simulink model "bench_flat"  (R2025b)
settings: Solver=ode4  StartTime=0.0  StopTime=inf  FixedStep=Ts_gcs  RelTol=1e-3
InitFcn:
  | bench_init_fcn(mocap);
undefined symbols (not defined in the file): mocap, Ts_gcs
libraries: instrumentseriallib x2, sldrtlib x1
Description:
  | Four-drone ground station of the FLATNESS variant (mirror of bench.slx).
  | MotiveMocapMulti streams every rigid body in mocap.streaming_ids, one gcu_flat instance
  | per entry (model argument drone_idx = slice of the shared traj built by bench_init_fcn).
  | Each path packs its own 106-byte flat frame; the four frames are concatenated into one
  | 424-byte USB frame, and gcs_sender_flat forwards the freshest frame per id.
  | Swarm mode: params; ref = swarm_precompute(...); init_trajectory_swarm(id) per drone; Run.
  | Evaluation: flight_evaluation_flat(id).
settings Model: DataDictionary=project.sldd  SimulationMode=accelerator  Creator=Nick  LastModifiedBy=Rakete
settings SolverCC: AutoInsertRateTranBlk=on

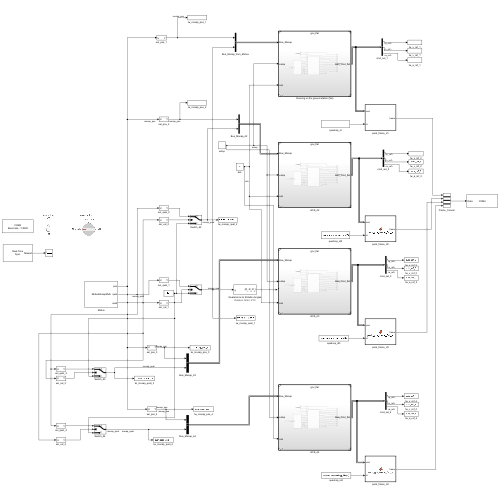
[thumbnail: Simulink's stored preview of the top-level diagram]
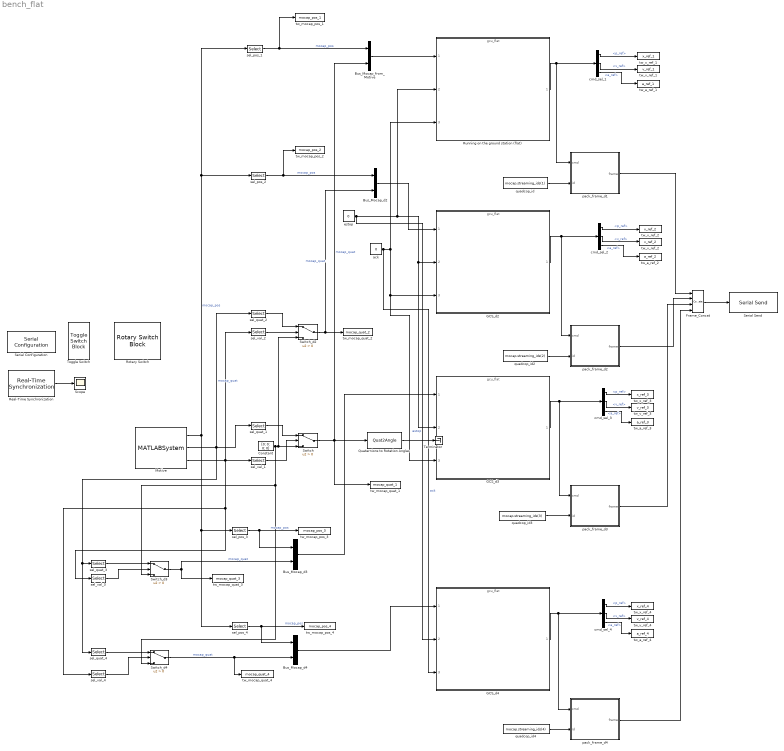
== system bench_flat ==
  Bus_Mocap_d2 : BusCreator  Inputs=2  OutDataTypeStr=Bus: Bus_Mocap
  Bus_Mocap_d3 : BusCreator  Inputs=2  OutDataTypeStr=Bus: Bus_Mocap
  Bus_Mocap_d4 : BusCreator  Inputs=2  OutDataTypeStr=Bus: Bus_Mocap
  Bus_Mocap_from_Motive : BusCreator  Inputs=2  OutDataTypeStr=Bus: Bus_Mocap
  Constant : Constant  Value=[0; 0; 0; 0]
  Frame_Concat : Concatenate  NumInputs=4
  GCS_d2 : ModelReference  ModelNameDialog=gcu_flat  ParameterArgumentNames=drone_idx  ParameterArgumentValues=2  UsingDefaultArgumentValue=0  SimulationMode=Normal  ModelReferenceVersion=1.330
  GCS_d3 : ModelReference  ModelNameDialog=gcu_flat  ParameterArgumentNames=drone_idx  ParameterArgumentValues=3  UsingDefaultArgumentValue=0  SimulationMode=Normal  ModelReferenceVersion=1.330
  GCS_d4 : ModelReference  ModelNameDialog=gcu_flat  ParameterArgumentNames=drone_idx  ParameterArgumentValues=4  UsingDefaultArgumentValue=0  SimulationMode=Normal  ModelReferenceVersion=1.330
  Motive : MATLABSystem  System=MotiveMocapMulti  HostIP=mocap.host_ip  ClientIP=mocap.client_ip  StreamingIDs=mocap.streaming_ids  SampleTimeSec=Ts_gcs  Verbose=on
      mask Type: MotiveMocapMulti
  Quaternions to Rotation Angles : Quat2Angle
      settings: AttributesFormatString=Rotation Order: %<rotationOrder>
  Real-Time Synchronization : sldrtlib/Real-Time Synchronization  SampleTime=Ts_gcs  MaxMissedTicks=inf  ShowMissedTicks=on  YieldWhenWaiting=off
  Rotary Switch : RotarySwitchBlock
  Running on the ground station (flat) : ModelReference  ModelNameDialog=gcu_flat  ParameterArgumentNames=drone_idx  ParameterArgumentValues=1  UsingDefaultArgumentValue=0  SimulationMode=Normal  ModelReferenceVersion=1.330
  Scope : Scope
      settings: ActiveDisplayYMinimum=-1  ActiveDisplayYMaximum=1
  Serial Configuration : instrumentseriallib/Serial Configuration  Priority=-200000  PortSel=COM4  Port=COM4  ComPort=COM4  BaudRate=115200  DataBits=8  Parity=none  StopBits=1  ByteOrder=little-endian  FlowControl=none  Timeout=10  SimulateUsing=Interpreted execution  BlockInModel=on  aMode=1
      settings: LibrarySourceBlock=c2000lib/Host Communication/Serial Configuration
  Serial Send : instrumentseriallib/Serial Send  Priority=1  PortSel=COM4  Port=COM4  ComPort=COM4  Header=[]  Terminator=<none>  CustomTerminator=[]  EnableBlockingMode=on  SimulateUsing=Interpreted execution  BlockInModel=on  aMode=1
      settings: LibrarySourceBlock=c2000lib/Host Communication/Serial Send
  Switch : Switch  Criteria=u2 > Threshold  SaturateOnIntegerOverflow=off  InputSameDT=off
  Switch_d2 : Switch  Criteria=u2 > Threshold  SaturateOnIntegerOverflow=off  InputSameDT=off
  Switch_d3 : Switch  Criteria=u2 > Threshold  SaturateOnIntegerOverflow=off  InputSameDT=off
  Switch_d4 : Switch  Criteria=u2 > Threshold  SaturateOnIntegerOverflow=off  InputSameDT=off
  Terminator : Terminator
  Toggle Switch : ToggleSwitchBlock
  ack : Constant  Value=0  OutDataTypeStr=boolean
  cmd_sel_{1..4} (4 alike) : BusSelector  OutputSignals=p_ref,v_ref,a_ref
  estop : Constant  Value=0  OutDataTypeStr=uint8
  pack_frame_d1 : MATLAB Function  TreatAsAtomicUnit=on
  pack_frame_d2 : MATLAB Function  TreatAsAtomicUnit=on
  pack_frame_d3 : MATLAB Function  TreatAsAtomicUnit=on
  pack_frame_d4 : MATLAB Function  TreatAsAtomicUnit=on
  quadcop_id : Constant  Value=mocap.streaming_ids(1)  OutDataTypeStr=uint8
  quadcop_id2 : Constant  Value=mocap.streaming_ids(2)  OutDataTypeStr=uint8
  quadcop_id3 : Constant  Value=mocap.streaming_ids(3)  OutDataTypeStr=uint8
  quadcop_id4 : Constant  Value=mocap.streaming_ids(4)  OutDataTypeStr=uint8
  sel_pos_1 : Selector  NumberOfDimensions=2  IndexOptions=Select all,Index vector (dialog)  Indices=1,1  OutputSizes=1
  sel_pos_2 : Selector  NumberOfDimensions=2  IndexOptions=Select all,Index vector (dialog)  Indices=1,2  OutputSizes=1
  sel_pos_3 : Selector  NumberOfDimensions=2  IndexOptions=Select all,Index vector (dialog)  Indices=1,3  OutputSizes=1
  sel_pos_4 : Selector  NumberOfDimensions=2  IndexOptions=Select all,Index vector (dialog)  Indices=1,4  OutputSizes=1
  sel_quat_1 : Selector  NumberOfDimensions=2  IndexOptions=Select all,Index vector (dialog)  Indices=1,1  OutputSizes=1
  sel_quat_2 : Selector  NumberOfDimensions=2  IndexOptions=Select all,Index vector (dialog)  Indices=1,2  OutputSizes=1
  sel_quat_3 : Selector  NumberOfDimensions=2  IndexOptions=Select all,Index vector (dialog)  Indices=1,3  OutputSizes=1
  sel_quat_4 : Selector  NumberOfDimensions=2  IndexOptions=Select all,Index vector (dialog)  Indices=1,4  OutputSizes=1
  sel_val_1 : Selector  IndexOptions=Index vector (dialog)  Indices=1  OutputSizes=1
  sel_val_2 : Selector  IndexOptions=Index vector (dialog)  Indices=2  OutputSizes=1
  sel_val_3 : Selector  IndexOptions=Index vector (dialog)  Indices=3  OutputSizes=1
  sel_val_4 : Selector  IndexOptions=Index vector (dialog)  Indices=4  OutputSizes=1
  tw_a_ref_1 : ToWorkspace  VariableName=a_ref_1  SaveFormat=Timeseries  SampleTime=Ts_gcs
  tw_a_ref_2 : ToWorkspace  VariableName=a_ref_2  SaveFormat=Timeseries  SampleTime=Ts_gcs
  tw_a_ref_3 : ToWorkspace  VariableName=a_ref_3  SaveFormat=Timeseries  SampleTime=Ts_gcs
  tw_a_ref_4 : ToWorkspace  VariableName=a_ref_4  SaveFormat=Timeseries  SampleTime=Ts_gcs
  tw_mocap_pos_1 : ToWorkspace  VariableName=mocap_pos_1  SaveFormat=Timeseries  SampleTime=Ts_gcs
  tw_mocap_pos_2 : ToWorkspace  VariableName=mocap_pos_2  SaveFormat=Timeseries  SampleTime=Ts_gcs
  tw_mocap_pos_3 : ToWorkspace  VariableName=mocap_pos_3  SaveFormat=Timeseries  SampleTime=Ts_gcs
  tw_mocap_pos_4 : ToWorkspace  VariableName=mocap_pos_4  SaveFormat=Timeseries  SampleTime=Ts_gcs
  tw_mocap_quat_1 : ToWorkspace  VariableName=mocap_quat_1  SaveFormat=Timeseries  SampleTime=Ts_gcs
  tw_mocap_quat_2 : ToWorkspace  VariableName=mocap_quat_2  SaveFormat=Timeseries  SampleTime=Ts_gcs
  tw_mocap_quat_3 : ToWorkspace  VariableName=mocap_quat_3  SaveFormat=Timeseries  SampleTime=Ts_gcs
  tw_mocap_quat_4 : ToWorkspace  VariableName=mocap_quat_4  SaveFormat=Timeseries  SampleTime=Ts_gcs
  tw_v_ref_1 : ToWorkspace  VariableName=v_ref_1  SaveFormat=Timeseries  SampleTime=Ts_gcs
  tw_v_ref_2 : ToWorkspace  VariableName=v_ref_2  SaveFormat=Timeseries  SampleTime=Ts_gcs
  tw_v_ref_3 : ToWorkspace  VariableName=v_ref_3  SaveFormat=Timeseries  SampleTime=Ts_gcs
  tw_v_ref_4 : ToWorkspace  VariableName=v_ref_4  SaveFormat=Timeseries  SampleTime=Ts_gcs
  tw_x_ref_1 : ToWorkspace  VariableName=x_ref_1  SaveFormat=Timeseries  SampleTime=Ts_gcs
  tw_x_ref_2 : ToWorkspace  VariableName=x_ref_2  SaveFormat=Timeseries  SampleTime=Ts_gcs
  tw_x_ref_3 : ToWorkspace  VariableName=x_ref_3  SaveFormat=Timeseries  SampleTime=Ts_gcs
  tw_x_ref_4 : ToWorkspace  VariableName=x_ref_4  SaveFormat=Timeseries  SampleTime=Ts_gcs
  wires:
  sel_val_1/1 -> Switch/2
  Motive/3 -> sel_val_3/1, sel_val_4/1, sel_val_1/1, sel_val_2/1
  Motive/1 -> sel_pos_3/1, sel_pos_4/1, sel_pos_2/1, sel_pos_1/1  "mocap_pos"
  Motive/2 -> sel_quat_3/1, sel_quat_4/1, sel_quat_1/1, sel_quat_2/1  "mocap_quat"
  quadcop_id2/1 -> pack_frame_d2/2(id)
  Real-Time Synchronization/1 -> Scope/1
  sel_pos_1/1 -> tw_mocap_pos_1/1, Bus_Mocap_from_Motive/1  "mocap_pos"
  sel_val_2/1 -> Switch_d2/2
  Switch_d2/1 -> tw_mocap_quat_2/1, Bus_Mocap_d2/2  "mocap_quat"
  sel_quat_1/1 -> Switch/1
  sel_quat_2/1 -> Switch_d2/1
  sel_pos_2/1 -> Bus_Mocap_d2/1, tw_mocap_pos_2/1  "mocap_pos"
  Constant/1 -> Switch_d3/3, Switch_d4/3, Switch/3, Switch_d2/3
  GCS_d2/1 -> pack_frame_d2/1(cmd), cmd_sel_2/1
  Switch/1 -> Quaternions to Rotation Angles/1, tw_mocap_quat_1/1, Bus_Mocap_from_Motive/2  "mocap_quat"
  Bus_Mocap_from_Motive/1 -> Running on the ground station (flat)/1
  pack_frame_d1/1(frame) -> Frame_Concat/1
  Bus_Mocap_d2/1 -> GCS_d2/1
  estop/1 -> GCS_d3/2, GCS_d2/2, Running on the ground station (flat)/2, GCS_d4/2  "estop"
  ack/1 -> GCS_d3/3, GCS_d2/3, Running on the ground station (flat)/3, GCS_d4/3  "ack"
  Running on the ground station (flat)/1 -> pack_frame_d1/1(cmd), cmd_sel_1/1
  Quaternions to Rotation Angles/1 -> Terminator/1
  quadcop_id/1 -> pack_frame_d1/2(id)
  cmd_sel_1/1 -> tw_x_ref_1/1  "<p_ref>"
  cmd_sel_1/2 -> tw_v_ref_1/1  "<v_ref>"
  cmd_sel_2/1 -> tw_x_ref_2/1  "<p_ref>"
  cmd_sel_2/2 -> tw_v_ref_2/1  "<v_ref>"
  pack_frame_d2/1(frame) -> Frame_Concat/2
  Frame_Concat/1 -> Serial Send/1
  sel_pos_3/1 -> Bus_Mocap_d3/1, tw_mocap_pos_3/1  "mocap_pos"
  sel_quat_3/1 -> Switch_d3/1
  sel_val_3/1 -> Switch_d3/2
  Switch_d3/1 -> Bus_Mocap_d3/2, tw_mocap_quat_3/1  "mocap_quat"
  Bus_Mocap_d3/1 -> GCS_d3/1
  GCS_d3/1 -> pack_frame_d3/1(cmd), cmd_sel_3/1
  quadcop_id3/1 -> pack_frame_d3/2(id)
  pack_frame_d3/1(frame) -> Frame_Concat/3
  cmd_sel_3/1 -> tw_x_ref_3/1  "<p_ref>"
  cmd_sel_3/2 -> tw_v_ref_3/1  "<v_ref>"
  sel_quat_4/1 -> Switch_d4/1
  sel_val_4/1 -> Switch_d4/2
  sel_pos_4/1 -> Bus_Mocap_d4/1, tw_mocap_pos_4/1  "mocap_pos"
  Switch_d4/1 -> tw_mocap_quat_4/1, Bus_Mocap_d4/2  "mocap_quat"
  Bus_Mocap_d4/1 -> GCS_d4/1
  GCS_d4/1 -> pack_frame_d4/1(cmd), cmd_sel_4/1
  quadcop_id4/1 -> pack_frame_d4/2(id)
  pack_frame_d4/1(frame) -> Frame_Concat/4
  cmd_sel_4/1 -> tw_x_ref_4/1  "<p_ref>"
  cmd_sel_4/2 -> tw_v_ref_4/1  "<v_ref>"
  cmd_sel_1/3 -> tw_a_ref_1/1  "<a_ref>"
  cmd_sel_2/3 -> tw_a_ref_2/1  "<a_ref>"
  cmd_sel_3/3 -> tw_a_ref_3/1  "<a_ref>"
  cmd_sel_4/3 -> tw_a_ref_4/1  "<a_ref>"

== matlab function bench_flat/pack_frame_d2 ==
  data: cmd input Bus: Bus_Cmd_flat; frame output uint8 size=[1 106]; id input uint8 size=[1 1]
function frame = pack_gcs_frame_flat_sl(cmd, id)
%#codegen
% WRAPPER -- haelt KEINE Logik. Single Source of Truth ist
% scripts\functions\pack_gcs_frame_flat.m; dieser Block ruft sie nur auf.
% Name MUSS abweichen (_sl), sonst schattet er die externe Funktion.
frame = pack_gcs_frame_flat(cmd, id);
end

== matlab function bench_flat/pack_frame_d3 ==
  data: cmd input Bus: Bus_Cmd_flat; frame output uint8 size=[1 106]; id input uint8 size=[1 1]
function frame = pack_gcs_frame_flat_sl(cmd, id)
%#codegen
% WRAPPER -- haelt KEINE Logik. Single Source of Truth ist
% scripts\functions\pack_gcs_frame_flat.m; dieser Block ruft sie nur auf.
% Name MUSS abweichen (_sl), sonst schattet er die externe Funktion.
frame = pack_gcs_frame_flat(cmd, id);
end

== matlab function bench_flat/pack_frame_d4 ==
  data: cmd input Bus: Bus_Cmd_flat; frame output uint8 size=[1 106]; id input uint8 size=[1 1]
function frame = pack_gcs_frame_flat_sl(cmd, id)
%#codegen
% WRAPPER -- haelt KEINE Logik. Single Source of Truth ist
% scripts\functions\pack_gcs_frame_flat.m; dieser Block ruft sie nur auf.
% Name MUSS abweichen (_sl), sonst schattet er die externe Funktion.
frame = pack_gcs_frame_flat(cmd, id);
end

== matlab function bench_flat/pack_frame_d1 ==
  data: cmd input Bus: Bus_Cmd_flat; frame output uint8 size=[1 106]; id input uint8 size=[1 1]
function frame = pack_gcs_frame_flat_sl(cmd, id)
%#codegen
% WRAPPER -- haelt KEINE Logik. Single Source of Truth ist
% scripts\functions\pack_gcs_frame_flat.m; dieser Block ruft sie nur auf.
% Name MUSS abweichen (_sl), sonst schattet er die externe Funktion.
frame = pack_gcs_frame_flat(cmd, id);
end
